simulink model "BRO_piston_MOD"  (R2020b)
settings: Solver=FixedStepAuto  StartTime=0.0  StopTime=time_max  FixedStep=.1  RelTol=1e-3
values from neighbouring files (symbols this model uses):
  A_mem = 30    [BRO_parameters_MOD.m]    (also in Copy_of_BRO_parameters_MOD.m; Large2.m = 29.6; Parameters_test2.m = 40.88; Small_Ref.m = 7.4)
  A_p = 0.25*pi*d_p^2    (= 0.00810731966556)    [BRO_parameters_MOD.m]    (also in Copy_of_BRO_parameters_MOD.m; Large2.m = 0.2105152; Parameters_test2.m = 1; Small_Ref.m = 0.03684016)
  A_w = 2/3600*1e-3    (= 5.55555555556e-07)    [BRO_parameters_MOD.m]    (also in Copy_of_BRO_parameters_MOD.m; Large2.m = 5.56e-12; Parameters_test2.m = 5.56e-07; Small_Ref.m = 5.56e-12)
  b = i*R*T*1e-2/M_NaCl*.93    (= 0.792350469684)    [BRO_parameters_MOD.m]    (also in Copy_of_BRO_parameters_MOD.m; Large2.m = 81215.9231426; Parameters_test2.m = 0.812159231426; Small_Ref.m = 81215.9231426)
  C_f_i = 35    [BRO_parameters_MOD.m]    (also in Copy_of_BRO_parameters_MOD.m; Large2.m; Parameters_test2.m; Small_Ref.m)
  D = 1.47e-9    (= 1.47e-09)    [BRO_parameters_MOD.m]    (also in Copy_of_BRO_parameters_MOD.m; Large2.m; Parameters_test2.m; Small_Ref.m)
  D_h = 2*t    (= 0.0014224)    [BRO_parameters_MOD.m]    (also in Copy_of_BRO_parameters_MOD.m; Large2.m; Parameters_test2.m = 0.056; Small_Ref.m)
  eta_cp = 0.65    [BRO_parameters_MOD.m]    (also in Copy_of_BRO_parameters_MOD.m; Large2.m; Parameters_test2.m; Small_Ref.m)
  eta_hp = 0.85    [BRO_parameters_MOD.m]    (also in Copy_of_BRO_parameters_MOD.m; Large2.m = 1; Parameters_test2.m; Small_Ref.m)
  L_mem = 0.96    [BRO_parameters_MOD.m]    (also in Copy_of_BRO_parameters_MOD.m; Large2.m; Parameters_test2.m = 1.016; Small_Ref.m)
  nu = 8.56e-7    (= 8.56e-07)    [BRO_parameters_MOD.m]    (also in Copy_of_BRO_parameters_MOD.m; Large2.m; Parameters_test2.m; Small_Ref.m)
  rho_f = 1025    [BRO_parameters_MOD.m]    (also in Copy_of_BRO_parameters_MOD.m; Large2.m; Parameters_test2.m; Small_Ref.m)
  Sc = nu/D    (= 582.31292517)    [BRO_parameters_MOD.m]    (also in Copy_of_BRO_parameters_MOD.m; Large2.m; Parameters_test2.m; Small_Ref.m)
  V_dot_cp = V_dot_hpp*(1-RR_pass)/RR_pass    (= 0.0135)    [BRO_parameters_MOD.m]    (also in Copy_of_BRO_parameters_MOD.m = 0.0015)
  V_dot_hpp = n_series * n_parallel * J_w*A_mem*(1e-3)/3600    (= 0.0015)    [BRO_parameters_MOD.m]    (also in Copy_of_BRO_parameters_MOD.m = 0.000166666666667)
  V_mem = A_mem*t/2    (= 0.010668)    [BRO_parameters_MOD.m]    (also in Copy_of_BRO_parameters_MOD.m; Large2.m = 0.01052576; Parameters_test2.m = 0.57232; Small_Ref.m = 0.00263144)
  V_tank_i = A_p*L_max    (= 0.00494222206813)    [BRO_parameters_MOD.m]    (also in Copy_of_BRO_parameters_MOD.m; Large2.m = 0.2105152; Parameters_test2.m = 4.57856; Small_Ref.m = 0.03684016)
settings Model: Creator=abhimanyu_das  LastModifiedBy=9alan

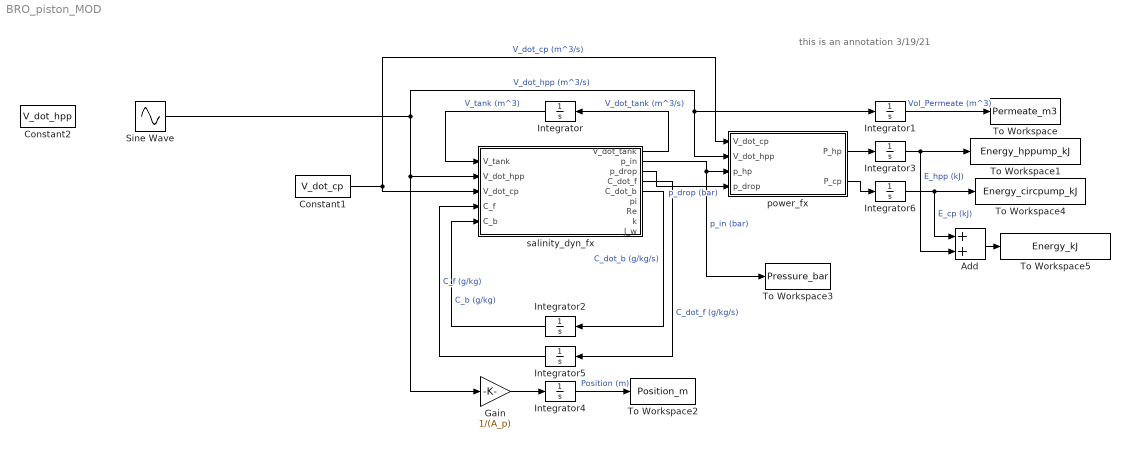
== system BRO_piston_MOD ==
  note: this is an annotation 3/19/21
  Add : Sum
  Constant1 : Constant  Value=V_dot_cp
  Constant2 : Constant  Value=V_dot_hpp
  Gain : Gain  Gain=1/(A_p)
  Integrator : Integrator  InitialCondition=V_tank_i
  Integrator{1,3..4,6} (4 alike) : Integrator
  Integrator2 : Integrator  InitialCondition=C_f_i
  Integrator5 : Integrator  InitialCondition=C_f_i
  Sine Wave : Sin  Amplitude=V_dot_hpp/4  Bias=V_dot_hpp  Frequency=.79  SampleTime=0
  To Workspace : ToWorkspace  VariableName=Permeate_m3  SaveFormat=Timeseries  SampleTime=-1
  To Workspace1 : ToWorkspace  VariableName=Energy_hppump_kJ  SaveFormat=Timeseries  SampleTime=-1
  To Workspace2 : ToWorkspace  VariableName=Position_m  SaveFormat=Timeseries  SampleTime=-1
  To Workspace3 : ToWorkspace  VariableName=Pressure_bar  SaveFormat=Timeseries  SampleTime=-1
  To Workspace4 : ToWorkspace  VariableName=Energy_circpump_kJ  SaveFormat=Timeseries  SampleTime=-1
  To Workspace5 : ToWorkspace  VariableName=Energy_kJ  SaveFormat=Timeseries  SampleTime=-1
  power_fx : MATLAB Function  TreatAsAtomicUnit=on
  salinity_dyn_fx : MATLAB Function  TreatAsAtomicUnit=on
  wires:
  salinity_dyn_fx/1(V_dot_tank) -> Integrator/1  "V_dot_tank (m^3/s)"
  Integrator/1 -> salinity_dyn_fx/1(V_tank)  "V_tank (m^3)"
  salinity_dyn_fx/5(C_dot_b) -> Integrator2/1  "C_dot_b (g/kg/s)"
  salinity_dyn_fx/4(C_dot_f) -> Integrator5/1  "C_dot_f (g/kg/s)"
  Integrator5/1 -> salinity_dyn_fx/4(C_f)  "C_f (g/kg)"
  Sine Wave/1 -> salinity_dyn_fx/2(V_dot_hpp), Gain/1, Integrator1/1, power_fx/2(V_dot_hpp)  "V_dot_hpp (m^3/s)"
  salinity_dyn_fx/2(p_in) -> To Workspace3/1, power_fx/3(p_hp)  "p_in (bar)"
  salinity_dyn_fx/3(p_drop) -> power_fx/4(p_drop)  "p_drop (bar)"
  Constant1/1 -> power_fx/1(V_dot_cp), salinity_dyn_fx/3(V_dot_cp)  "V_dot_cp (m^3/s)"
  power_fx/1(P_hp) -> Integrator3/1
  Integrator3/1 -> Add/2, To Workspace1/1  "E_hpp (kJ)"
  Integrator1/1 -> To Workspace/1  "Vol_Permeate (m^3)"
  Gain/1 -> Integrator4/1
  Integrator4/1 -> To Workspace2/1  "Position (m)"
  Integrator2/1 -> salinity_dyn_fx/5(C_b)  "C_b (g/kg)"
  power_fx/2(P_cp) -> Integrator6/1
  Integrator6/1 -> Add/1, To Workspace4/1  "E_cp (kJ)"
  Add/1 -> To Workspace5/1

== matlab function BRO_piston_MOD/power_fx ==
  data: V_dot_cp input; V_dot_hpp input; p_hp input; p_drop input; P_hp output; eta_cp parameter; eta_hp parameter; P_cp output
function [P_hp,P_cp] = Power(V_dot_cp, V_dot_hpp, p_hp, p_drop, eta_cp, eta_hp)

P_hp = V_dot_hpp*p_hp*100/eta_hp;       %high pressure pump power consumption [kW]   %is this quite right? Are we actually assuming the inlet to the HPP is atmospheric?
P_cp = V_dot_cp*p_drop*100/eta_cp;     %circulation pump power consumption [kW]

%Power = P_hp + P_cp;

== matlab function BRO_piston_MOD/salinity_dyn_fx ==
  data: V_tank input; V_dot_tank output; p_in output; p_drop output; V_dot_hpp input; V_dot_cp input; C_f input; C_b input; V_mem parameter; C_dot_f output; C_dot_b output; A_mem parameter; rho_f parameter; A_w parameter; D parameter; D_h parameter; b parameter; Sc parameter; nu parameter; L_mem parameter; pi output; Re output; k output; J_w output
function [V_dot_tank, p_in, p_drop, C_dot_f, C_dot_b,pi,Re,k,J_w] = Salinity_dynamics(V_tank, V_dot_hpp, V_dot_cp, C_f, C_b, V_mem, A_mem, rho_f, A_w, D, D_h, b, Sc, nu, L_mem)

V_dot_f = V_dot_hpp + V_dot_cp;
V_dot_b = V_dot_cp;
V_dot_tank = -V_dot_hpp;

%EQN SHEET
%rate of change of amt of salt in pist tank (first eqn) 
C_dot_f = (-V_dot_f*C_f + V_dot_b*C_b - C_f*V_dot_tank)/V_tank; 

%rate of change of amt of salt in top part of mem module (Cmem eqn) 
C_dot_b = 2*(V_dot_f*C_f - V_dot_b*C_b)/V_mem - C_dot_f;

V_dot = 0.5*(V_dot_f + V_dot_b);        %Average flow rate on feed side (m^3/s)
u_avg = V_dot*4*L_mem/(D_h*A_mem);      %Average velocity on feed side (m/s)
Re = u_avg*D_h/nu;                      %Reynolds number                     
Sh = .20*(Re^.57*Sc^.4);       %Sherwood number  https://www.sciencedirect.com/science/article/pii/S0011916420313035?via%3Dihub

k = Sh*D/D_h;                           %Mass transfer coefficient [m/s]

C_f_avg = 0.5*(C_f+C_b);                %Average bulk salinity on feed side (g/kg)
J_w = V_dot_hpp/A_mem;                  %instantaneous flux (m/s)
pi = b*C_f_avg*exp(J_w/k);              %Feed side osmotic pressure (bar)  USE this ConcPolarization eqn
%pi = b*C_f_avg;    %do not use
%pi = SW_OsmPress(300,'K',C_f_avg*exp(J_w/k),'ppt')*10 %bar

p_in = J_w/A_w + pi;                %hi p pump pressure (bar)    
f = 3.23*Re^-0.3;                  %friction factor
p_drop = f*L_mem*rho_f*u_avg^2*1e-5/(2*D_h); %Pressure drop across a membrane module (bar)
